simulink model "EC_segun_atributo"  (R2023b)
settings: Solver=VariableStepAuto  StartTime=0.0  StopTime=20  RelTol=1e-3
undefined symbols (not defined in the file or in its folder): m
settings Model: Creator=anruk  LastModifiedBy=anruk

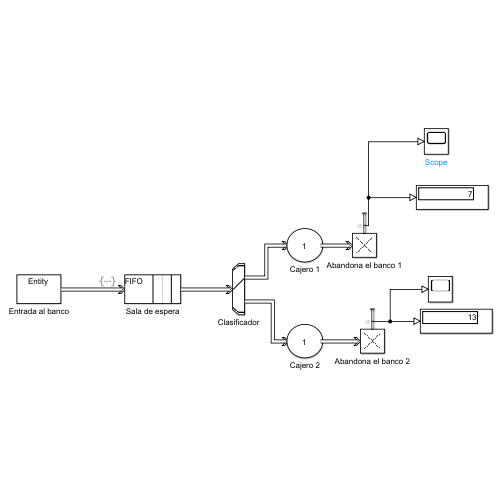
[thumbnail: Simulink's stored preview of the top-level diagram]
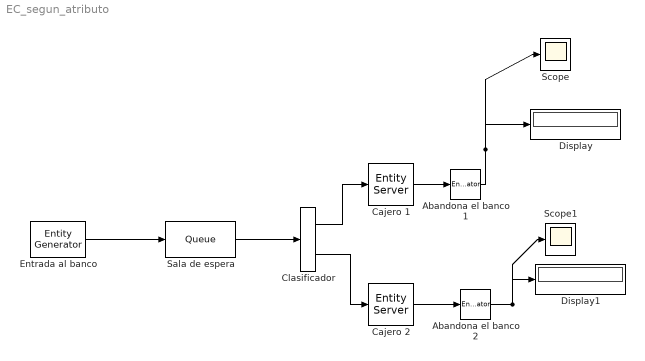
== system EC_segun_atributo ==
  Abandona el banco 1 : EntityTerminator  InputPortMessageModes=m  NumberEntitiesArrived=on
      settings: OutputPortMap=o0
  Abandona el banco 2 : EntityTerminator  InputPortMessageModes=m  NumberEntitiesArrived=on
      settings: OutputPortMap=o0
  Cajero 1 : EntityServer  InputPortMessageModes=m  OutputPortMessageModes=m  Capacity=1
  Cajero 2 : EntityServer  InputPortMessageModes=m  OutputPortMessageModes=m  Capacity=1
  Clasificador : EntityOutputSwitch  InputPortMessageModes=m  OutputPortMessageModes=m,m  SwitchingCriterion=From attribute  SwitchAttributeName=TransaccionTipo
  Display : Display
  Display1 : Display
  Entrada al banco : EntityGenerator  OutputPortMessageModes=m  AttributeName=TransaccionTipo  AttributeInitialValue=0  EntityType=Structured  EntityTypeName=Entity
  Sala de espera : Queue  InputPortMessageModes=m  OutputPortMessageModes=m  EntryAction=entity.TransaccionTipo = randi([1,2]);
  Scope : Scope
  Scope1 : Scope
  wires:
  Entrada al banco/1 -> Sala de espera/1
  Sala de espera/1 -> Clasificador/1
  Clasificador/1 -> Cajero 1/1
  Clasificador/2 -> Cajero 2/1
  Cajero 2/1 -> Abandona el banco 2/1
  Cajero 1/1 -> Abandona el banco 1/1
  Abandona el banco 1/1 -> Scope/1, Display/1
  Abandona el banco 2/1 -> Scope1/1, Display1/1
